simulink model "Untitled"  (R2021a)
settings: Solver=VariableStepAuto  StartTime=0.0  StopTime=10.0  RelTol=1e-3
model workspace (MAT data in the model file):
  teta = [-1.5 0.54 2 -1.8]
values from neighbouring files (symbols this model uses):
  A = [1 5 0.6]    [Untitled.m]
  B = [1 0.2 0.1]    [Untitled.m]    (also in efge.m = zeros(d,1))
  C = [0 -4.8 -0.5]    [Untitled.m]
settings Model: OrderedModelArguments=off  Creator=Krisz  LastModifiedBy=Krisz

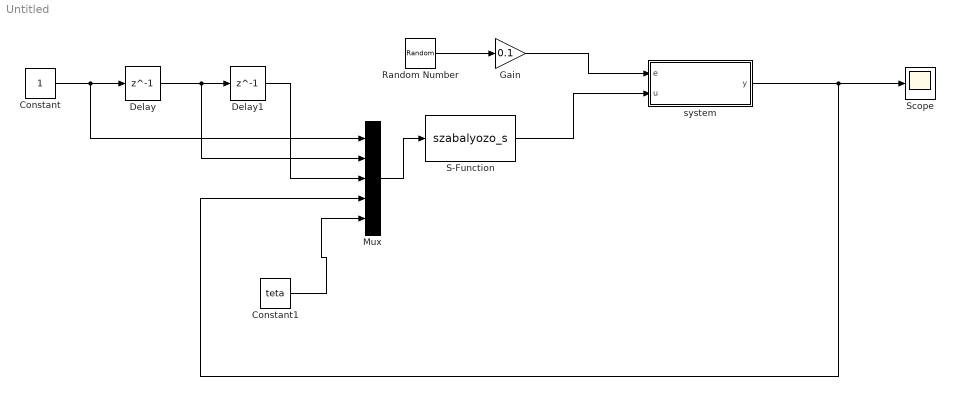
== system Untitled ==
  Constant : Constant
  Constant1 : Constant  Value=teta
  Delay : Delay  DelayLength=1
  Delay1 : Delay  DelayLength=1
  Gain : Gain  Gain=0.1
  Mux : Mux  Inputs=5
  Random Number : RandomNumber  Variance=0.01  SampleTime=0.1
  S-Function : S-Function  FunctionName=szabalyozo_s  SFunctionDeploymentMode=off  EnableBusSupport=off
  Scope : Scope
  system : Subsystem  mask{A=A, B=B, C=C}
  wires:
  Random Number/1 -> Gain/1
  Gain/1 -> system/1(e)
  S-Function/1 -> system/2(u)
  Constant1/1 -> Mux/5
  system/1(y) -> Mux/4, Scope/1
  Mux/1 -> S-Function/1
  Delay/1 -> Mux/2, Delay1/1
  Delay1/1 -> Mux/3
  Constant/1 -> Delay/1, Mux/1

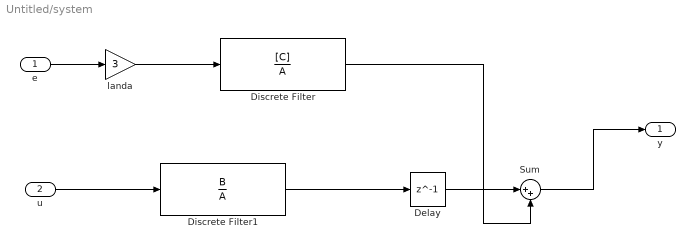
== system Untitled/system ==
  e : Inport
  u : Inport  Port=2
  Delay : Delay  DelayLength=1  InitialCondition=0
  Discrete Filter : DiscreteFilter  Numerator=[C]  Denominator=A
  Discrete Filter1 : DiscreteFilter  Numerator=B  Denominator=A
  Sum : Sum  Inputs=|++
  landa : Gain  Gain=3
  y : Outport
  wires:
  Discrete Filter1/1 -> Delay/1
  Delay/1 -> Sum/1
  Discrete Filter/1 -> Sum/2
  landa/1 -> Discrete Filter/1
  u/1 -> Discrete Filter1/1
  e/1 -> landa/1
  Sum/1 -> y/1
